simulink model "target_driver_2022_Ctrl_v_2_4_landing_2017a"  (R2024b)
settings: Solver=FixedStepDiscrete  StartTime=0.0  StopTime=13  FixedStep=0.0001  RelTol=1e-3  EnableMultiTasking=on
values from neighbouring files (symbols this model uses):
  A = gamma_2*gamma_3*Thrust_desired    [force2voltage.m]
  a2_lb = -0.25    [target_driver_setup_2022_Ctrl_V_2_4.m]    (also in target_driver_setup_2022_Ctrl_V_2_4_geometric.m; target_driver_setup_mpc_12msdelay.m; target_driver_setup_mpc_andWLQP.m)
  a2_openloop = -0    (= 0)    [target_driver_setup_2022_Ctrl_V_2_4.m]    (also in target_driver_setup_2022_Ctrl_V_2_4_geometric.m; target_driver_setup_mpc_12msdelay.m; target_driver_setup_mpc_andWLQP.m)
  a2_ub = 0.25    [target_driver_setup_2022_Ctrl_V_2_4.m]    (also in target_driver_setup_2022_Ctrl_V_2_4_geometric.m; target_driver_setup_mpc_12msdelay.m; target_driver_setup_mpc_andWLQP.m)
  adaptive_flag = 0    [target_driver_setup_2022_Ctrl_V_2_4.m]    (also in target_driver_setup_2022_Ctrl_V_2_4_geometric.m; target_driver_setup_mpc_12msdelay.m = 1; target_driver_setup_mpc_andWLQP.m = 1)
  adaptive_gain = [gamma_adaptive, adaptive_roll_limit, adaptive_pitch_limit, adaptive_yaw_limit, c_2_adaptive, gamma_lateral_adaptive, adaptive_x_limit, adaptive_y_limit, adaptive_z_limit, c_1_adaptive]    [target_driver_setup_2022_Ctrl_V_2_4.m]    (also in target_driver_setup_2022_Ctrl_V_2_4_geometric.m; target_driver_setup_mpc_12msdelay.m; target_driver_setup_mpc_andWLQP.m)
  adaptive_lateral_flag = 0    [target_driver_setup_2022_Ctrl_V_2_4.m]    (also in target_driver_setup_2022_Ctrl_V_2_4_geometric.m; target_driver_setup_mpc_12msdelay.m = 1; target_driver_setup_mpc_andWLQP.m = 1)
  adaptive_pitch_init = 0    [target_driver_setup_2022_Ctrl_V_2_4.m]    (also in target_driver_setup_2022_Ctrl_V_2_4_geometric.m; target_driver_setup_mpc_12msdelay.m; target_driver_setup_mpc_andWLQP.m)
  adaptive_pitch_limit = 0.1/(scale^2)    (= 1e-07)    [target_driver_setup_2022_Ctrl_V_2_4.m]    (also in target_driver_setup_2022_Ctrl_V_2_4_geometric.m = 3e-07; target_driver_setup_mpc_12msdelay.m; target_driver_setup_mpc_andWLQP.m)
  adaptive_pitch_limit_low = -adaptive_pitch_limit    (= -1e-07)    [target_driver_setup_2022_Ctrl_V_2_4.m]    (also in target_driver_setup_2022_Ctrl_V_2_4_geometric.m = -3e-07; target_driver_setup_mpc_12msdelay.m; target_driver_setup_mpc_andWLQP.m)
  adaptive_roll_init = 0    [target_driver_setup_2022_Ctrl_V_2_4.m]    (also in target_driver_setup_2022_Ctrl_V_2_4_geometric.m; target_driver_setup_mpc_12msdelay.m; target_driver_setup_mpc_andWLQP.m)
  adaptive_roll_limit = 0.3/(scale^2)    (= 3e-07)    [target_driver_setup_2022_Ctrl_V_2_4.m]    (also in target_driver_setup_2022_Ctrl_V_2_4_geometric.m; target_driver_setup_mpc_12msdelay.m; target_driver_setup_mpc_andWLQP.m)
  adaptive_roll_limit_low = -adaptive_roll_limit    (= -3e-07)    [target_driver_setup_2022_Ctrl_V_2_4.m]    (also in target_driver_setup_2022_Ctrl_V_2_4_geometric.m; target_driver_setup_mpc_12msdelay.m; target_driver_setup_mpc_andWLQP.m)
  adaptive_x_init = 0    [target_driver_setup_2022_Ctrl_V_2_4.m]    (also in target_driver_setup_2022_Ctrl_V_2_4_geometric.m; target_driver_setup_mpc_12msdelay.m; target_driver_setup_mpc_andWLQP.m)
  adaptive_x_limit = 0.15/(scale)    (= 0.00015)    [target_driver_setup_2022_Ctrl_V_2_4.m]    (also in target_driver_setup_2022_Ctrl_V_2_4_geometric.m = 7.5e-05; target_driver_setup_mpc_12msdelay.m; target_driver_setup_mpc_andWLQP.m)
  adaptive_x_limit_low = -adaptive_x_limit    (= -0.00015)    [target_driver_setup_2022_Ctrl_V_2_4.m]    (also in target_driver_setup_2022_Ctrl_V_2_4_geometric.m = -7.5e-05; target_driver_setup_mpc_12msdelay.m; target_driver_setup_mpc_andWLQP.m)
  adaptive_y_init = 0    [target_driver_setup_2022_Ctrl_V_2_4.m]    (also in target_driver_setup_2022_Ctrl_V_2_4_geometric.m; target_driver_setup_mpc_12msdelay.m; target_driver_setup_mpc_andWLQP.m)
  adaptive_y_limit = 0.15/(scale)    (= 0.00015)    [target_driver_setup_2022_Ctrl_V_2_4.m]    (also in target_driver_setup_2022_Ctrl_V_2_4_geometric.m = 7.5e-05; target_driver_setup_mpc_12msdelay.m; target_driver_setup_mpc_andWLQP.m)
  adaptive_y_limit_low = -adaptive_y_limit    (= -0.00015)    [target_driver_setup_2022_Ctrl_V_2_4.m]    (also in target_driver_setup_2022_Ctrl_V_2_4_geometric.m = -7.5e-05; target_driver_setup_mpc_12msdelay.m; target_driver_setup_mpc_andWLQP.m)
  adaptive_yaw_init = 0    [target_driver_setup_2022_Ctrl_V_2_4.m]    (also in target_driver_setup_2022_Ctrl_V_2_4_geometric.m; target_driver_setup_mpc_12msdelay.m; target_driver_setup_mpc_andWLQP.m)
  adaptive_yaw_limit = 0.035/(scale^2)    (= 3.5e-08)    [target_driver_setup_2022_Ctrl_V_2_4.m]    (also in target_driver_setup_2022_Ctrl_V_2_4_geometric.m; target_driver_setup_mpc_12msdelay.m; target_driver_setup_mpc_andWLQP.m)
  adaptive_yaw_limit_low = -adaptive_yaw_limit    (= -3.5e-08)    [target_driver_setup_2022_Ctrl_V_2_4.m]    (also in target_driver_setup_2022_Ctrl_V_2_4_geometric.m; target_driver_setup_mpc_12msdelay.m; target_driver_setup_mpc_andWLQP.m)
  adaptive_z_init = 0/scale    (= 0)    [target_driver_setup_2022_Ctrl_V_2_4.m]    (also in target_driver_setup_2022_Ctrl_V_2_4_geometric.m; target_driver_setup_mpc_12msdelay.m; target_driver_setup_mpc_andWLQP.m)
  adaptive_z_limit = 0.20/(scale)    (= 0.0002)    [target_driver_setup_2022_Ctrl_V_2_4.m]    (also in target_driver_setup_2022_Ctrl_V_2_4_geometric.m = 0.0008; target_driver_setup_mpc_12msdelay.m = 0.0008; target_driver_setup_mpc_andWLQP.m = 0.0008)
  adaptive_z_limit_low = -adaptive_z_limit/1    (= -0.0002)    [target_driver_setup_2022_Ctrl_V_2_4.m]    (also in target_driver_setup_2022_Ctrl_V_2_4_geometric.m = -0.0008; target_driver_setup_mpc_12msdelay.m = -0.0008; target_driver_setup_mpc_andWLQP.m = -0.0008)
  att_s = 500    [target_driver_setup_2022_Ctrl_V_2_4.m]    (also in target_driver_setup_2022_Ctrl_V_2_4_geometric.m; target_driver_setup_mpc_12msdelay.m; target_driver_setup_mpc_andWLQP.m)
  b_1_d_desired = [1,0,0]    [target_driver_setup_2022_Ctrl_V_2_4.m]    (also in target_driver_setup_2022_Ctrl_V_2_4_geometric.m; target_driver_setup_mpc_12msdelay.m; target_driver_setup_mpc_andWLQP.m)
  closedloop_flag = 1    [target_driver_setup_2022_Ctrl_V_2_4.m]    (also in target_driver_setup_2022_Ctrl_V_2_4_geometric.m = 0; target_driver_setup_mpc_12msdelay.m = 0; target_driver_setup_mpc_andWLQP.m = 0)
  control_gain = [k_x,k_v, k_R, k_Omega, k_z, k_vz, k_Rx]    [target_driver_setup_2022_Ctrl_V_2_4.m]    (also in target_driver_setup_2022_Ctrl_V_2_4_geometric.m = [k_x,k_v,k_R,k_Omega_pitch,k_Omega_roll,k_z,k_vz,k_Rx]; target_driver_setup_mpc_12msdelay.m = [k_x, k_v, k_R, k_Omega, k_z, k_vz, k_Rx,                  k; target_driver_setup_mpc_andWLQP.m = [k_x, k_v, k_R, k_Omega, k_z, k_vz, k_Rx,                  k)
  delay = delay-vicon_sample_cycle/2    [target_driver_setup_2022_Ctrl_V_2_4.m]    (also in target_driver_setup_2022_Ctrl_V_2_4_geometric.m; target_driver_setup_mpc_12msdelay.m; target_driver_setup_mpc_andWLQP.m)
  drv_amp = abs((vleft_p2p-vright_p2p))/2+min(vleft_p2p,vright_p2p)    [Wing_traj_to_Voltage.m]    (also in force2voltage.m; target_driver_setup_2022_Ctrl_V_2_4.m = 160; target_driver_setup_2022_Ctrl_V_2_4_geometric.m = 110; target_driver_setup_mpc_12msdelay.m = 150)
  drv_bias = max_drv_bias    (= 300)    [target_driver_setup_2022_Ctrl_V_2_4.m]    (also in target_driver_setup_2022_Ctrl_V_2_4_geometric.m = 200; target_driver_setup_mpc_12msdelay.m = 200; target_driver_setup_mpc_andWLQP.m = 200)
  drv_pitch_left = vleft_pitch    [Wing_traj_to_Voltage.m]    (also in force2voltage.m = 0; target_driver_setup_2022_Ctrl_V_2_4.m = 0; target_driver_setup_2022_Ctrl_V_2_4_geometric.m = 9.05; target_driver_setup_mpc_12msdelay.m = 9.05)
  drv_pitch_right = vright_pitch    [Wing_traj_to_Voltage.m]    (also in force2voltage.m = 0; target_driver_setup_2022_Ctrl_V_2_4.m = 0; target_driver_setup_2022_Ctrl_V_2_4_geometric.m = 9.05; target_driver_setup_mpc_12msdelay.m = 9.05)
  drv_roll = (vleft_p2p-vright_p2p)/4    [Wing_traj_to_Voltage.m]    (also in force2voltage.m; target_driver_setup_2022_Ctrl_V_2_4.m = -2; target_driver_setup_2022_Ctrl_V_2_4_geometric.m = -0.001; target_driver_setup_mpc_12msdelay.m = -0.001)
  f_fin = f    (= 155)    [target_driver_setup_2022_Ctrl_V_2_4.m]    (also in target_driver_setup_2022_Ctrl_V_2_4_geometric.m; target_driver_setup_mpc_12msdelay.m; target_driver_setup_mpc_andWLQP.m)
  f_int = f    (= 155)    [target_driver_setup_2022_Ctrl_V_2_4.m]    (also in target_driver_setup_2022_Ctrl_V_2_4_geometric.m; target_driver_setup_mpc_12msdelay.m; target_driver_setup_mpc_andWLQP.m)
  g = 9.8    [target_driver_setup_2022_Ctrl_V_2_4.m]    (also in target_driver_setup_2022_Ctrl_V_2_4_geometric.m; target_driver_setup_mpc_12msdelay.m; target_driver_setup_mpc_andWLQP.m = 9.81; test_full_attitude_mpc.m = 9.81)
  I_moment_vec = [Ixx, Iyy, Izz]    [target_driver_setup_2022_Ctrl_V_2_4.m]    (also in target_driver_setup_2022_Ctrl_V_2_4_geometric.m; target_driver_setup_mpc_12msdelay.m; target_driver_setup_mpc_andWLQP.m)
  landing_flag = 0    [target_driver_setup_2022_Ctrl_V_2_4.m]    (also in target_driver_setup_2022_Ctrl_V_2_4_geometric.m; target_driver_setup_mpc_12msdelay.m; target_driver_setup_mpc_andWLQP.m)
  landing_parameter = [start_delay+T,transition_rate, rising_time, falling_time, landing_rising_time, landing_z_decrease, landing_y_decrease, landing_x_decrease]    [target_driver_setup_2022_Ctrl_V_2_4.m]    (also in target_driver_setup_2022_Ctrl_V_2_4_geometric.m; target_driver_setup_mpc_12msdelay.m; target_driver_setup_mpc_andWLQP.m)
  low_bound = -8    [target_driver_setup_2022_Ctrl_V_2_4.m]    (also in target_driver_setup_2022_Ctrl_V_2_4_geometric.m = -5; target_driver_setup_mpc_12msdelay.m = -10; target_driver_setup_mpc_andWLQP.m = -10)
  low_bound_eR = -0.8    [target_driver_setup_2022_Ctrl_V_2_4.m]    (also in target_driver_setup_2022_Ctrl_V_2_4_geometric.m = -1.2; target_driver_setup_mpc_12msdelay.m = -1.2; target_driver_setup_mpc_andWLQP.m = -1.2)
  low_bound_vx = -0.5    [target_driver_setup_2022_Ctrl_V_2_4.m]    (also in target_driver_setup_2022_Ctrl_V_2_4_geometric.m; target_driver_setup_mpc_12msdelay.m; target_driver_setup_mpc_andWLQP.m)
  low_bound_vy = -0.5    [target_driver_setup_2022_Ctrl_V_2_4.m]    (also in target_driver_setup_2022_Ctrl_V_2_4_geometric.m; target_driver_setup_mpc_12msdelay.m; target_driver_setup_mpc_andWLQP.m)
  low_bound_vz = -0.5    [target_driver_setup_2022_Ctrl_V_2_4.m]    (also in target_driver_setup_2022_Ctrl_V_2_4_geometric.m; target_driver_setup_mpc_12msdelay.m; target_driver_setup_mpc_andWLQP.m)
  low_bound_x = -0.06    [target_driver_setup_2022_Ctrl_V_2_4.m]    (also in target_driver_setup_2022_Ctrl_V_2_4_geometric.m = -0.1; target_driver_setup_mpc_12msdelay.m = -0.6; target_driver_setup_mpc_andWLQP.m = -0.6)
  low_bound_y = -0.06    [target_driver_setup_2022_Ctrl_V_2_4.m]    (also in target_driver_setup_2022_Ctrl_V_2_4_geometric.m; target_driver_setup_mpc_12msdelay.m = -0.6; target_driver_setup_mpc_andWLQP.m = -0.6)
  low_bound_z = -0.04    [target_driver_setup_2022_Ctrl_V_2_4.m]    (also in target_driver_setup_2022_Ctrl_V_2_4_geometric.m; target_driver_setup_mpc_12msdelay.m = -0.1; target_driver_setup_mpc_andWLQP.m = -0.1)
  m = t <= t_zoom    [plot_roll_torque_cmd_vs_actual.m]    (also in plot_roll_torque_cmd_vs_actual_flightlog.m = t >= t0 & t <= t1; target_driver_setup_2022_Ctrl_V_2_4.m = 0.000124; target_driver_setup_2022_Ctrl_V_2_4_geometric.m = 8.5655e-05; target_driver_setup_mpc_12msdelay.m = 8.5655e-05)
  params_vec = [params_opt.delta_1, params_opt.delta_2, params_opt.delta_3,      params_opt.gamma_1, params_opt.gamma_2_1, params_opt.gamma_3,      params_opt.eta, params_opt.nu, params_opt.mu]'    [force2voltage_tuningSandbox.m]    (also in target_driver_setup_2022_Ctrl_V_2_4.m = [params_opt.delta_1, params_opt.delta_2, params_opt.delta_3,; target_driver_setup_2022_Ctrl_V_2_4_geometric.m = [params_opt.delta_1, params_opt.delta_2, params_opt.delta_3,; target_driver_setup_mpc_12msdelay.m = [params_opt.delta_1, params_opt.delta_2, params_opt.delta_3,; target_driver_setup_mpc_andWLQP.m = [params_opt.delta_1, params_opt.delta_2, params_opt.delta_3,)
  phase = 0    [target_driver_setup_2022_Ctrl_V_2_4.m]    (also in target_driver_setup_2022_Ctrl_V_2_4_geometric.m; target_driver_setup_mpc_12msdelay.m; target_driver_setup_mpc_andWLQP.m)
  r_desired = [default_x, default_y,z_desired]    [target_driver_setup_2022_Ctrl_V_2_4.m]    (also in target_driver_setup_2022_Ctrl_V_2_4_geometric.m; target_driver_setup_mpc_12msdelay.m; target_driver_setup_mpc_andWLQP.m)
  roll_offset_angle = 0    [target_driver_setup_2022_Ctrl_V_2_4.m]    (also in target_driver_setup_2022_Ctrl_V_2_4_geometric.m; target_driver_setup_mpc_12msdelay.m; target_driver_setup_mpc_andWLQP.m)
  running_time = start_delay+total_T    (= 8.5)    [target_driver_setup_2022_Ctrl_V_2_4.m]    (also in target_driver_setup_2022_Ctrl_V_2_4_geometric.m = 10; target_driver_setup_mpc_12msdelay.m = 0.5; target_driver_setup_mpc_andWLQP.m = 10)
  running_time_control = start_delay_control+total_T+0.0    (= 8.6)    [target_driver_setup_2022_Ctrl_V_2_4.m]    (also in target_driver_setup_2022_Ctrl_V_2_4_geometric.m = 10; target_driver_setup_mpc_12msdelay.m = 0.5; target_driver_setup_mpc_andWLQP.m = 10)
  start_delay = 2.0    (= 2)    [target_driver_setup_2022_Ctrl_V_2_4.m]    (also in target_driver_setup_2022_Ctrl_V_2_4_geometric.m = 0; target_driver_setup_mpc_12msdelay.m = 0; target_driver_setup_mpc_andWLQP.m = 0)
  start_delay_control = start_delay + ramp_delay    (= 2.1)    [target_driver_setup_2022_Ctrl_V_2_4.m]    (also in target_driver_setup_2022_Ctrl_V_2_4_geometric.m = 0; target_driver_setup_mpc_12msdelay.m = 0; target_driver_setup_mpc_andWLQP.m = 0)
  T = 0.5    [target_driver_setup_2022_Ctrl_V_2_4.m]    (also in target_driver_setup_2022_Ctrl_V_2_4_geometric.m = 10; target_driver_setup_mpc_12msdelay.m; target_driver_setup_mpc_andWLQP.m = 10; test_full_attitude_mpc.m = T0 + nu(1))
  task_flag = 0    [target_driver_setup_2022_Ctrl_V_2_4.m]    (also in target_driver_setup_2022_Ctrl_V_2_4_geometric.m; target_driver_setup_mpc_12msdelay.m; target_driver_setup_mpc_andWLQP.m)
  task_parameter = [radius_ref, frequency_ref, radius_ratio, lissajous_ratio, lissajous_delta, lissajous_amplitude_ratio,z_radius_ratio]    [target_driver_setup_2022_Ctrl_V_2_4.m]    (also in target_driver_setup_2022_Ctrl_V_2_4_geometric.m; target_driver_setup_mpc_12msdelay.m; target_driver_setup_mpc_andWLQP.m)
  upp_bound = 8    [target_driver_setup_2022_Ctrl_V_2_4.m]    (also in target_driver_setup_2022_Ctrl_V_2_4_geometric.m = 5; target_driver_setup_mpc_12msdelay.m = 10; target_driver_setup_mpc_andWLQP.m = 10)
  upp_bound_eR = 0.8    [target_driver_setup_2022_Ctrl_V_2_4.m]    (also in target_driver_setup_2022_Ctrl_V_2_4_geometric.m = 1.2; target_driver_setup_mpc_12msdelay.m = 1.2; target_driver_setup_mpc_andWLQP.m = 1.2)
  upp_bound_vx = 0.5    [target_driver_setup_2022_Ctrl_V_2_4.m]    (also in target_driver_setup_2022_Ctrl_V_2_4_geometric.m; target_driver_setup_mpc_12msdelay.m; target_driver_setup_mpc_andWLQP.m)
  upp_bound_vy = 0.5    [target_driver_setup_2022_Ctrl_V_2_4.m]    (also in target_driver_setup_2022_Ctrl_V_2_4_geometric.m; target_driver_setup_mpc_12msdelay.m; target_driver_setup_mpc_andWLQP.m)
  upp_bound_vz = 0.5    [target_driver_setup_2022_Ctrl_V_2_4.m]    (also in target_driver_setup_2022_Ctrl_V_2_4_geometric.m; target_driver_setup_mpc_12msdelay.m; target_driver_setup_mpc_andWLQP.m)
  upp_bound_x = 0.06    [target_driver_setup_2022_Ctrl_V_2_4.m]    (also in target_driver_setup_2022_Ctrl_V_2_4_geometric.m = 0.1; target_driver_setup_mpc_12msdelay.m = 0.6; target_driver_setup_mpc_andWLQP.m = 0.6)
  upp_bound_y = 0.06    [target_driver_setup_2022_Ctrl_V_2_4.m]    (also in target_driver_setup_2022_Ctrl_V_2_4_geometric.m; target_driver_setup_mpc_12msdelay.m = 0.6; target_driver_setup_mpc_andWLQP.m = 0.6)
  upp_bound_z = 0.04    [target_driver_setup_2022_Ctrl_V_2_4.m]    (also in target_driver_setup_2022_Ctrl_V_2_4_geometric.m; target_driver_setup_mpc_12msdelay.m = 0.1; target_driver_setup_mpc_andWLQP.m = 0.1)
undefined symbols (not defined in the file or in its folder): Com1, DiscIntNeverNeededParam, left_mapping, left_mapping_F_to_Phi, lp_den, lp_num, none, right_mapping, right_mapping_F_to_Phi, vlp_den, vlp_num
libraries: simulink x32, xpcseriallib x6, xpcnilib x3, xpcutilitieslib x3
(part 2 of 7)

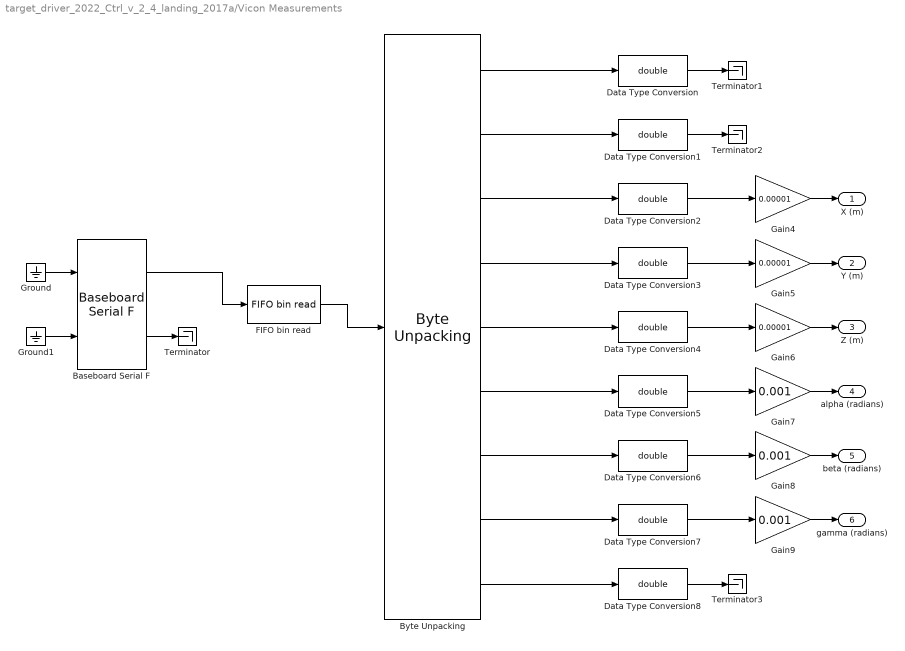
== system target_driver_2022_Ctrl_v_2_4_landing_2017a/Vicon Measurements ==
  Baseboard Serial F : xpcseriallib/Mainboard/Baseboard Serial F  group=FIFO Setup  port=1  irqnum=4  saddr1=0x3f8  saddr2=0x3e8  config=Com1/none  baud1=115200  parity1=None  ndata1=8  nstop1=1  fifomode1=16 deep  rlevel1=half full  automode1=on  xmtfifosize1=1024  xmtdatatype1=8 bit int null terminated  rcvfifosize1=1024  baud2=115200  parity2=None  ndata2=8  nstop2=1  fifomode2=16 deep  rlevel2=half full  automode2=off  xmtfifosize2=1024  xmtdatatype2=8 bit uint null terminated  rcvfifosize2=1024
      settings: SourceProductName=Simulink Real-Time
  "Byte Unpacking " : xpcutilitieslib/Byte Unpacking   MaskUnpackedDataTypes={'uint8','int16','int16','int16','int16','int16','int16','int16','uint8'}  MaskUnpackedDataSizes={[1] [1] [1] [1] [1] [1] [1] [1] [1]}  MaskAlignment=1
      settings: SourceProductName=Simulink Real-Time
  Data Type Conversion{,1..8} (9 alike) : DataTypeConversion  OutDataTypeStr=double  SaturateOnIntegerOverflow=off  RndMeth=Floor
  "FIFO bin read " : xpcseriallib/FIFO bin read   header=[128,127,127]  lengths=[15]  hold=Hold last output if no new data  enable=off  maxsize=15  outputtype=8 bit uint null terminated  sampletime=0.0001
      settings: SourceProductName=Simulink Real-Time
  Gain4 : Gain  Gain=0.00001
  Gain5 : Gain  Gain=0.00001
  Gain6 : Gain  Gain=0.00001
  Gain7 : Gain  Gain=0.001
  Gain8 : Gain  Gain=0.001
  Gain9 : Gain  Gain=0.001
  Ground : Ground
  Ground1 : Ground
  Terminator{,1..3} (4 alike) : Terminator
  X (m) : Outport
  Y (m) : Outport  Port=2
  Z (m) : Outport  Port=3
  alpha (radians) : Outport  Port=4
  beta (radians) : Outport  Port=5
  gamma (radians) : Outport  Port=6
  wires:
  Baseboard Serial F/1 -> "FIFO bin read "/1
  Baseboard Serial F/2 -> Terminator/1
  Ground1/1 -> Baseboard Serial F/2
  Ground/1 -> Baseboard Serial F/1
  "Byte Unpacking "/1 -> Data Type Conversion/1
  "Byte Unpacking "/2 -> Data Type Conversion1/1
  "Byte Unpacking "/3 -> Data Type Conversion2/1
  "Byte Unpacking "/4 -> Data Type Conversion3/1
  "FIFO bin read "/1 -> "Byte Unpacking "/1
  "Byte Unpacking "/8 -> Data Type Conversion7/1
  "Byte Unpacking "/7 -> Data Type Conversion6/1
  "Byte Unpacking "/5 -> Data Type Conversion4/1
  "Byte Unpacking "/6 -> Data Type Conversion5/1
  Data Type Conversion3/1 -> Gain5/1
  Data Type Conversion4/1 -> Gain6/1
  Data Type Conversion5/1 -> Gain7/1
  Data Type Conversion6/1 -> Gain8/1
  Data Type Conversion7/1 -> Gain9/1
  "Byte Unpacking "/9 -> Data Type Conversion8/1
  Gain4/1 -> X (m)/1
  Data Type Conversion2/1 -> Gain4/1
  Gain5/1 -> Y (m)/1
  Gain6/1 -> Z (m)/1
  Gain7/1 -> alpha (radians)/1
  Gain8/1 -> beta (radians)/1
  Gain9/1 -> gamma (radians)/1
  Data Type Conversion/1 -> Terminator1/1
  Data Type Conversion1/1 -> Terminator2/1
  Data Type Conversion8/1 -> Terminator3/1

== system target_driver_2022_Ctrl_v_2_4_landing_2017a/Vicon Post Processing ==
  note: Process Vicon data
      |
      | 1) Generate Raw rotation matrix
      | 2) Flag the update of new vicon data
      | 3) Count the number of samples before new update
      |
      | By Patrick 2021 Mar
  alpha : Inport
  beta : Inport  Port=2
  gamma : Inport  Port=3
  Raw rotation matrix : Subsystem
  Vicon Validity check : Subsystem
  Vicon correction : MATLAB Function  TreatAsAtomicUnit=on
  roll_offset_angle : Constant  Value=roll_offset_angle  SampleTime=-1
  "Vicon Update Flag " : Outport
  Raw Rotation Matrix : Outport  Port=2
  "Vicon Count " : Outport  Port=3
  wires:
  Vicon Validity check/2(Vicon Count) -> "Vicon Count "/1
  beta/1 -> Raw rotation matrix/2(beta)
  gamma/1 -> Raw rotation matrix/3(gamma)
  alpha/1 -> Raw rotation matrix/1(alpha)
  Vicon Validity check/1("Vicon Update flag ") -> "Vicon Update Flag "/1
  roll_offset_angle/1 -> Vicon correction/2(roll_offset_angle)
  Raw rotation matrix/1(R) -> Vicon correction/1(R_cur)
  Vicon correction/1(Rot_corrected_vec) -> Raw Rotation Matrix/1, Vicon Validity check/1("Rotation Matrix ")

== system target_driver_2022_Ctrl_v_2_4_landing_2017a/Vicon Post Processing1 ==
  note: Process Vicon data
      |
      | 1) Generate Raw rotation matrix
      | 2) Flag the update of new vicon data
      | 3) Count the number of samples before new update
      |
      | By Patrick 2021 Mar
  alpha : Inport
  beta : Inport  Port=2
  gamma : Inport  Port=3
  Raw rotation matrix : Subsystem
  Vicon Validity check : Subsystem
  Vicon correction : MATLAB Function  TreatAsAtomicUnit=on
  roll_offset_angle : Constant  Value=roll_offset_angle  SampleTime=-1
  "Vicon Update Flag " : Outport
  Raw Rotation Matrix : Outport  Port=2
  "Vicon Count " : Outport  Port=3
  wires:
  Vicon Validity check/2(Vicon Count) -> "Vicon Count "/1
  beta/1 -> Raw rotation matrix/2(beta)
  gamma/1 -> Raw rotation matrix/3(gamma)
  alpha/1 -> Raw rotation matrix/1(alpha)
  Vicon Validity check/1("Vicon Update flag ") -> "Vicon Update Flag "/1
  roll_offset_angle/1 -> Vicon correction/2(roll_offset_angle)
  Raw rotation matrix/1(R) -> Vicon correction/1(R_cur)
  Vicon correction/1(Rot_corrected_vec) -> Raw Rotation Matrix/1, Vicon Validity check/1("Rotation Matrix ")

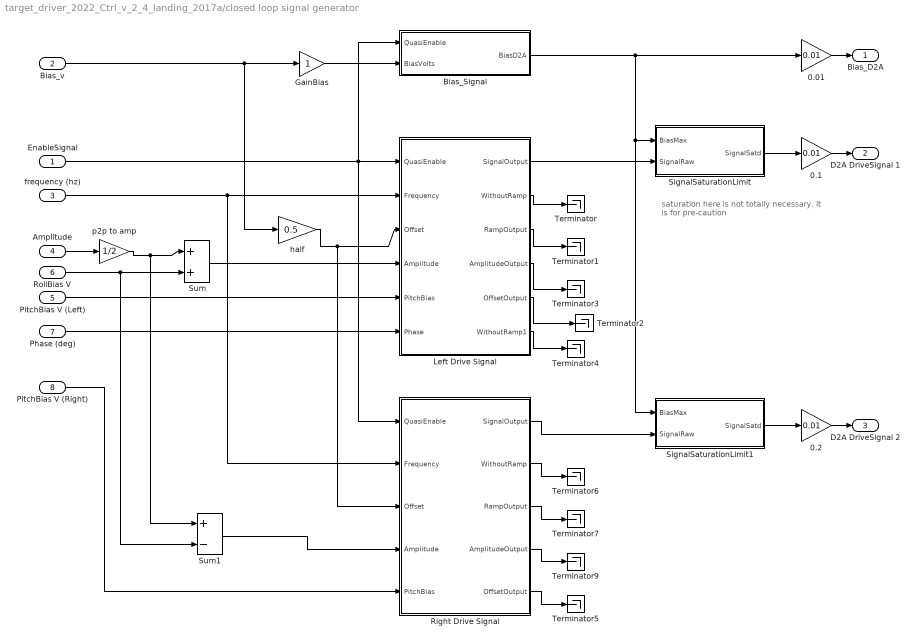
== system target_driver_2022_Ctrl_v_2_4_landing_2017a/closed loop signal generator ==
  note: saturation here is not totally necessary.
      | it is for pre-caution
  EnableSignal : Inport
  Bias_v : Inport  Port=2
  frequency (hz) : Inport  Port=3
  Amplitude : Inport  Port=4
  PitchBias V (Left) : Inport  Port=5
  RollBias V : Inport  Port=6
  Phase (deg) : Inport  Port=7
  PitchBias V (Right) : Inport  Port=8
  0.01 : Gain  Gain=0.01
  0.1 : Gain  Gain=0.01
  0.2 : Gain  Gain=0.01
  Bias_Signal : Subsystem
  GainBias : Gain
  "Left Drive Signal " : Subsystem
  Right Drive Signal : Subsystem
  SignalSaturationLimit : Subsystem
  SignalSaturationLimit1 : Subsystem
  Sum : Sum
  Sum1 : Sum  Inputs=+-
  Terminator{,1..7,9} (9 alike) : Terminator
  half : Gain  Gain=0.5
  p2p to amp : Gain  Gain=1/2
  Bias_D2A : Outport
  D2A DriveSignal 1 : Outport  Port=2
  D2A DriveSignal 2 : Outport  Port=3
  wires:
  Bias_Signal/1(BiasD2A) -> SignalSaturationLimit1/1(BiasMax), SignalSaturationLimit/1(BiasMax), 0.01/1
  half/1 -> "Left Drive Signal "/3(Offset), Right Drive Signal/3(Offset)
  Bias_v/1 -> GainBias/1, half/1
  EnableSignal/1 -> "Left Drive Signal "/1(QuasiEnable), Bias_Signal/1(QuasiEnable), Right Drive Signal/1(QuasiEnable)
  frequency (hz)/1 -> Right Drive Signal/2(Frequency), "Left Drive Signal "/2(Frequency)
  "Left Drive Signal "/2(WithoutRamp) -> Terminator/1
  "Left Drive Signal "/3(RampOutput) -> Terminator1/1
  "Left Drive Signal "/5(OffsetOutput) -> Terminator2/1
  SignalSaturationLimit/1(SignalSatd) -> 0.1/1
  GainBias/1 -> Bias_Signal/2(BiasVolts)
  Sum/1 -> "Left Drive Signal "/4(Amplitude)
  RollBias V/1 -> Sum/2, Sum1/2
  SignalSaturationLimit1/1(SignalSatd) -> 0.2/1
  Right Drive Signal/5(OffsetOutput) -> Terminator5/1
  Amplitude/1 -> p2p to amp/1
  p2p to amp/1 -> Sum/1, Sum1/1
  "Left Drive Signal "/4(AmplitudeOutput) -> Terminator3/1
  Right Drive Signal/2(WithoutRamp) -> Terminator6/1
  Right Drive Signal/3(RampOutput) -> Terminator7/1
  Right Drive Signal/4(AmplitudeOutput) -> Terminator9/1
  0.01/1 -> Bias_D2A/1
  0.1/1 -> D2A DriveSignal 1/1
  0.2/1 -> D2A DriveSignal 2/1
  Sum1/1 -> Right Drive Signal/4(Amplitude)
  Right Drive Signal/1(SignalOutput) -> SignalSaturationLimit1/2(SignalRaw)
  "Left Drive Signal "/1(SignalOutput) -> SignalSaturationLimit/2(SignalRaw)
  Phase (deg)/1 -> "Left Drive Signal "/6(Phase)
  "Left Drive Signal "/6(WithoutRamp1) -> Terminator4/1
  PitchBias V (Left)/1 -> "Left Drive Signal "/5(PitchBias)
  PitchBias V (Right)/1 -> Right Drive Signal/5(PitchBias)

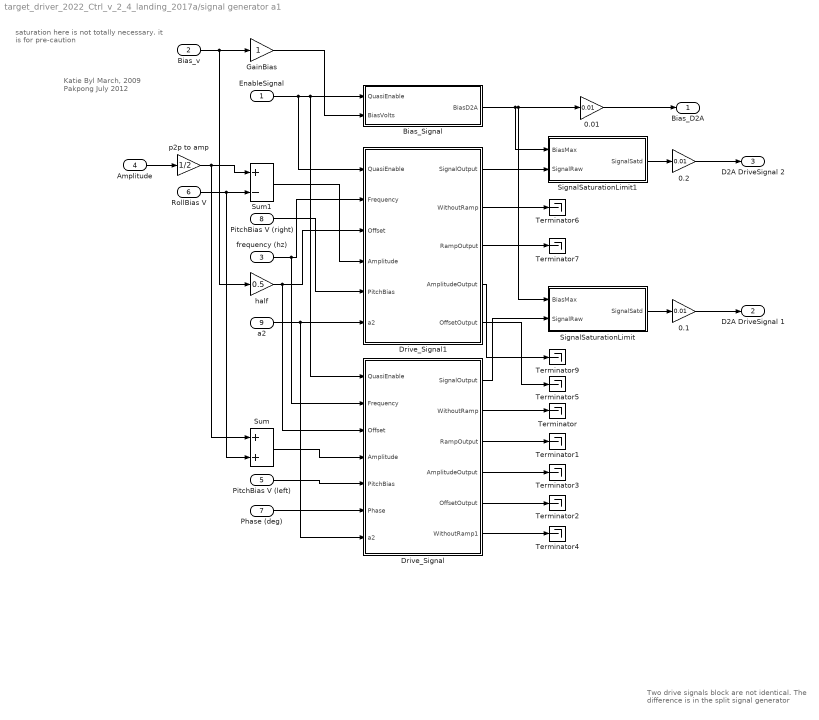
== system target_driver_2022_Ctrl_v_2_4_landing_2017a/signal generator a1 ==
  note: Katie Byl
      | March, 2009
      |
      | Pakpong
      | July 2012
  note: Two drive signals block are not identical.
      | The difference is in the split signal generator
  note: saturation here is not totally necessary.
      | it is for pre-caution
  EnableSignal : Inport
  Bias_v : Inport  Port=2
  frequency (hz) : Inport  Port=3
  Amplitude : Inport  Port=4
  PitchBias V (left) : Inport  Port=5
  RollBias V : Inport  Port=6
  Phase (deg) : Inport  Port=7
  PitchBias V (right) : Inport  Port=8
  a2 : Inport  Port=9
  0.01 : Gain  Gain=0.01
  0.1 : Gain  Gain=0.01
  0.2 : Gain  Gain=0.01
  Bias_Signal : Subsystem
  Drive_Signal : Subsystem
  Drive_Signal1 : Subsystem
  GainBias : Gain
  SignalSaturationLimit : Subsystem
  SignalSaturationLimit1 : Subsystem
  Sum : Sum
  Sum1 : Sum  Inputs=+-
  Terminator{,1..7,9} (9 alike) : Terminator
  half : Gain  Gain=0.5
  p2p to amp : Gain  Gain=1/2
  Bias_D2A : Outport
  D2A DriveSignal 1 : Outport  Port=2
  D2A DriveSignal 2 : Outport  Port=3
  wires:
  0.1/1 -> D2A DriveSignal 1/1
  0.2/1 -> D2A DriveSignal 2/1
  SignalSaturationLimit1/1(SignalSatd) -> 0.2/1
  0.01/1 -> Bias_D2A/1
  SignalSaturationLimit/1(SignalSatd) -> 0.1/1
  Drive_Signal/5(OffsetOutput) -> Terminator2/1
  GainBias/1 -> Bias_Signal/2(BiasVolts)
  Drive_Signal/1(SignalOutput) -> SignalSaturationLimit/2(SignalRaw)
  Drive_Signal1/5(OffsetOutput) -> Terminator5/1
  half/1 -> Drive_Signal1/3(Offset), Drive_Signal/3(Offset)
  Drive_Signal1/4(AmplitudeOutput) -> Terminator9/1
  Drive_Signal1/3(RampOutput) -> Terminator7/1
  PitchBias V (left)/1 -> Drive_Signal/5(PitchBias)
  Bias_Signal/1(BiasD2A) -> 0.01/1, SignalSaturationLimit/1(BiasMax), SignalSaturationLimit1/1(BiasMax)
  Drive_Signal1/2(WithoutRamp) -> Terminator6/1
  Drive_Signal/6(WithoutRamp1) -> Terminator4/1
  a2/1 -> Drive_Signal1/6(a2), Drive_Signal/7("a2 ")
  Drive_Signal/2(WithoutRamp) -> Terminator/1
  Phase (deg)/1 -> Drive_Signal/6(Phase)
  frequency (hz)/1 -> Drive_Signal/2(Frequency), Drive_Signal1/2(Frequency)
  RollBias V/1 -> Sum1/2, Sum/2
  Sum1/1 -> Drive_Signal1/4(Amplitude)
  Drive_Signal/4(AmplitudeOutput) -> Terminator3/1
  PitchBias V (right)/1 -> Drive_Signal1/5(PitchBias)
  EnableSignal/1 -> Bias_Signal/1(QuasiEnable), Drive_Signal/1(QuasiEnable), Drive_Signal1/1(QuasiEnable)
  Amplitude/1 -> p2p to amp/1
  Sum/1 -> Drive_Signal/4(Amplitude)
  Bias_v/1 -> half/1, GainBias/1
  Drive_Signal/3(RampOutput) -> Terminator1/1
  Drive_Signal1/1(SignalOutput) -> SignalSaturationLimit1/2(SignalRaw)
  p2p to amp/1 -> Sum1/1, Sum/1

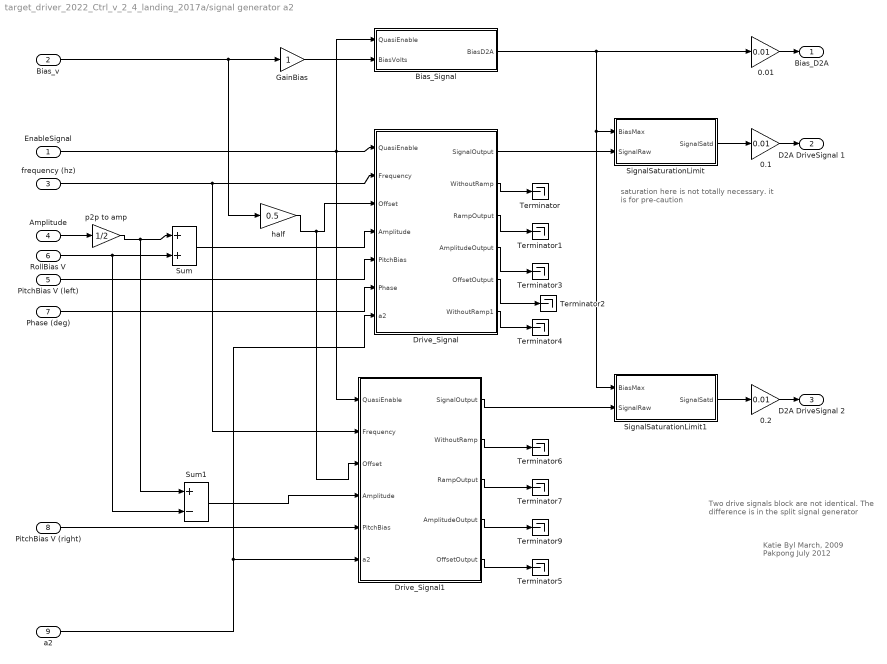
== system target_driver_2022_Ctrl_v_2_4_landing_2017a/signal generator a2 ==
  note: Katie Byl
      | March, 2009
      |
      | Pakpong
      | July 2012
  note: Two drive signals block are not identical.
      | The difference is in the split signal generator
  note: saturation here is not totally necessary.
      | it is for pre-caution
  EnableSignal : Inport
  Bias_v : Inport  Port=2
  frequency (hz) : Inport  Port=3
  Amplitude : Inport  Port=4
  PitchBias V (left) : Inport  Port=5
  RollBias V : Inport  Port=6
  Phase (deg) : Inport  Port=7
  PitchBias V (right) : Inport  Port=8
  a2 : Inport  Port=9
  0.01 : Gain  Gain=0.01
  0.1 : Gain  Gain=0.01
  0.2 : Gain  Gain=0.01
  Bias_Signal : Subsystem
  Drive_Signal : Subsystem
  Drive_Signal1 : Subsystem
  GainBias : Gain
  SignalSaturationLimit : Subsystem
  SignalSaturationLimit1 : Subsystem
  Sum : Sum
  Sum1 : Sum  Inputs=+-
  Terminator{,1..7,9} (9 alike) : Terminator
  half : Gain  Gain=0.5
  p2p to amp : Gain  Gain=1/2
  Bias_D2A : Outport
  D2A DriveSignal 1 : Outport  Port=2
  D2A DriveSignal 2 : Outport  Port=3
  wires:
  Bias_Signal/1(BiasD2A) -> SignalSaturationLimit1/1(BiasMax), SignalSaturationLimit/1(BiasMax), 0.01/1
  half/1 -> Drive_Signal/3(Offset), Drive_Signal1/3(Offset)
  Bias_v/1 -> GainBias/1, half/1
  EnableSignal/1 -> Drive_Signal/1(QuasiEnable), Bias_Signal/1(QuasiEnable), Drive_Signal1/1(QuasiEnable)
  frequency (hz)/1 -> Drive_Signal1/2(Frequency), Drive_Signal/2(Frequency)
  Drive_Signal/2(WithoutRamp) -> Terminator/1
  Drive_Signal/3(RampOutput) -> Terminator1/1
  Drive_Signal/5(OffsetOutput) -> Terminator2/1
  SignalSaturationLimit/1(SignalSatd) -> 0.1/1
  GainBias/1 -> Bias_Signal/2(BiasVolts)
  Sum/1 -> Drive_Signal/4(Amplitude)
  RollBias V/1 -> Sum/2, Sum1/2
  SignalSaturationLimit1/1(SignalSatd) -> 0.2/1
  Drive_Signal1/5(OffsetOutput) -> Terminator5/1
  Amplitude/1 -> p2p to amp/1
  p2p to amp/1 -> Sum/1, Sum1/1
  Drive_Signal/4(AmplitudeOutput) -> Terminator3/1
  Drive_Signal1/2(WithoutRamp) -> Terminator6/1
  Drive_Signal1/3(RampOutput) -> Terminator7/1
  Drive_Signal1/4(AmplitudeOutput) -> Terminator9/1
  0.01/1 -> Bias_D2A/1
  0.1/1 -> D2A DriveSignal 1/1
  0.2/1 -> D2A DriveSignal 2/1
  Sum1/1 -> Drive_Signal1/4(Amplitude)
  Drive_Signal1/1(SignalOutput) -> SignalSaturationLimit1/2(SignalRaw)
  Drive_Signal/1(SignalOutput) -> SignalSaturationLimit/2(SignalRaw)
  Phase (deg)/1 -> Drive_Signal/6(Phase)
  Drive_Signal/6(WithoutRamp1) -> Terminator4/1
  PitchBias V (left)/1 -> Drive_Signal/5(PitchBias)
  a2/1 -> Drive_Signal/7("a2 "), Drive_Signal1/6(a2)
  PitchBias V (right)/1 -> Drive_Signal1/5(PitchBias)

== system target_driver_2022_Ctrl_v_2_4_landing_2017a/timer1 ==
  SaturatingRamp : DiscreteIntegrator  gainval=1  SampleTime=-1  UpperSaturationLimit=1  LowerSaturationLimit=0  ICPrevOutput=DiscIntNeverNeededParam  ICPrevScaledInput=DiscIntNeverNeededParam
  constant : Constant
  time : Outport
  wires:
  SaturatingRamp/1 -> time/1
  constant/1 -> SaturatingRamp/1

== system target_driver_2022_Ctrl_v_2_4_landing_2017a/Desired attitude and normalized error/Geometric derivative for Rd in SO(3) ==
  note: First order geometric derivative Rd in SO(3)
      | Patrick 2021 Mar
  Previous Averaged Rotation M : Inport
  Vicon Count : Inport  Port=2
  Current Averaged Rotation M : Inport  Port=3
  "Vicon Update Flag " : Inport  Port=4
  Demux1 : Demux  Outputs=3
  Demux2 : Demux  Outputs=3
  Discrete Derivative : simulink/Discrete/Discrete Derivative  gainval=1.0  ICPrevScaledInput=0.0  OutMin=[]  OutMax=[]  OutDataType=fixdt(1, 16)  OutScaling=2^-10  DoSatur=off
  "First order geometric derivative in SO(3) " : MATLAB Function  TreatAsAtomicUnit=on
  Mux1 : Mux  Inputs=3
  Mux2 : Mux  Inputs=3
  Previous Omega_d : Delay  DelayLength=1  InitialCondition=0
  filtered derivative1 : Subsystem
  filtered derivative5 : Subsystem
  Filtered Geometric derivative dRd in SO(3) : Outport
  Filtered Geometric derivative ddRd in SO(3)1 : Outport  Port=2
  wires:
  Previous Omega_d/1 -> "First order geometric derivative in SO(3) "/3(omega_d_prev)
  Previous Averaged Rotation M/1 -> "First order geometric derivative in SO(3) "/1(R_prev)
  Demux2/1 -> Mux2/1
  Demux2/2 -> Mux2/2
  filtered derivative5/1(Out1) -> Discrete Derivative/1, Demux2/1
  Mux2/1 -> Filtered Geometric derivative dRd in SO(3)/1
  "First order geometric derivative in SO(3) "/1(omega_d) -> Previous Omega_d/1, filtered derivative5/1(In1)
  Demux2/3 -> Mux2/3
  Current Averaged Rotation M/1 -> "First order geometric derivative in SO(3) "/2(R_cur)
  Vicon Count/1 -> "First order geometric derivative in SO(3) "/5(count)
  "Vicon Update Flag "/1 -> "First order geometric derivative in SO(3) "/4(update)
  Demux1/3 -> Mux1/3
  Mux1/1 -> Filtered Geometric derivative ddRd in SO(3)1/1
  Demux1/2 -> Mux1/2
  filtered derivative1/1(Out1) -> Demux1/1
  Demux1/1 -> Mux1/1
  Discrete Derivative/1 -> filtered derivative1/1(In1)

== system target_driver_2022_Ctrl_v_2_4_landing_2017a/Desired attitude and normalized error/saturated normalized error observation ==
  p : Inport
  v : Inport  Port=2
  R : Inport  Port=3
  omega : Inport  Port=4
  "omega_desired " : Inport  Port=5
  R_desired : Inport  Port=6
  r_desired : Inport  Port=7
  "v_desired " : Inport  Port=8
  "Saturated angular velocity eOmega " : Subsystem
  Saturated normalized eR : Subsystem
  "saturated normalized altitude error " : Subsystem
  "Normalized omega error " : Outport
  Normalized eR : Outport  Port=2
  "Normalized position error " : Outport  Port=3
  Normalized velocity error : Outport  Port=4
  wires:
  omega/1 -> "Saturated angular velocity eOmega "/1(omega)
  v/1 -> "saturated normalized altitude error "/1(averaged velocity)
  p/1 -> "saturated normalized altitude error "/2(averaged position)
  Saturated normalized eR/1(normalized eR) -> Normalized eR/1
  R/1 -> "Saturated angular velocity eOmega "/3(R_cur), Saturated normalized eR/1(Current averaged rotation M)
  R_desired/1 -> "Saturated angular velocity eOmega "/4(R_desired), Saturated normalized eR/2(R_desired)
  "Saturated angular velocity eOmega "/1(Normalized angular velocity) -> "Normalized omega error "/1
  "omega_desired "/1 -> "Saturated angular velocity eOmega "/2("omega_desired ")
  "saturated normalized altitude error "/1(Position error) -> "Normalized position error "/1
  "saturated normalized altitude error "/2(velocity_error) -> Normalized velocity error/1
  "v_desired "/1 -> "saturated normalized altitude error "/4(v_desired)
  r_desired/1 -> "saturated normalized altitude error "/3("r_desired ")

== system target_driver_2022_Ctrl_v_2_4_landing_2017a/Geometric Controller/Attitude Adaptive ==
  e_R : Inport
  e_Omega : Inport  Port=2
  Enable : Inport  Port=3
  Adaptive_flag : Inport  Port=4
  adaptive_gain : Inport  Port=5
  Adaptive Control : MATLAB Function  TreatAsAtomicUnit=on
  Compare To Zero : simulink/Logic and Bit Operations/Compare To Zero  relop=>  OutDataTypeStr=uint8  ZeroCross=off
  "Integrator " : DiscreteIntegrator  InitialConditionSource=external  InitialCondition=adaptive_roll_init  SampleTime=-1  LimitOutput=on  UpperSaturationLimit=adaptive_roll_limit  LowerSaturationLimit=adaptive_roll_limit_low  ICPrevOutput=DiscIntNeverNeededParam  ICPrevScaledInput=DiscIntNeverNeededParam
  Integrator 1 : DiscreteIntegrator  InitialConditionSource=external  InitialCondition=adaptive_pitch_init  SampleTime=-1  LimitOutput=on  UpperSaturationLimit=adaptive_pitch_limit  LowerSaturationLimit=adaptive_pitch_limit_low  ICPrevOutput=DiscIntNeverNeededParam  ICPrevScaledInput=DiscIntNeverNeededParam
  Integrator 2 : DiscreteIntegrator  InitialConditionSource=external  InitialCondition=adaptive_yaw_init  SampleTime=-1  LimitOutput=on  UpperSaturationLimit=adaptive_yaw_limit  LowerSaturationLimit=adaptive_yaw_limit_low  ICPrevOutput=DiscIntNeverNeededParam  ICPrevScaledInput=DiscIntNeverNeededParam
  Mux : Mux  Inputs=3
  Product{1,5..10} (7 alike) : Product  RndMeth=Zero
  adaptive_pitch_init : Constant  Value=adaptive_pitch_init
  "adaptive_roll_init " : Constant  Value=adaptive_roll_init
  adaptive_yaw_init : Constant  Value=adaptive_yaw_init
  adaptive_roll : Outport
  adaptive_pitch : Outport  Port=2
  adaptive_yaw : Outport  Port=3
  adaptive_attitude_control : Outport  Port=4
  wires:
  Product5/1 -> "Integrator "/1
  Adaptive Control/1(der_adaptive_torque_roll) -> Product5/2
  Product6/1 -> Integrator 1/1
  Adaptive Control/2(der_adaptive_torque_pitch) -> Product6/2
  Product7/1 -> Integrator 2/1
  Product8/1 -> adaptive_roll/1
  Adaptive Control/3(der_adaptive_torque_yaw) -> Product7/2
  Product9/1 -> adaptive_pitch/1
  Product10/1 -> adaptive_yaw/1
  Adaptive_flag/1 -> Compare To Zero/1
  Compare To Zero/1 -> Product1/1, Product10/1, Product9/1, Product8/1
  Integrator 2/1 -> Mux/3, Product10/2, Adaptive Control/3(current_adaptive_yaw)
  Integrator 1/1 -> Product9/2, Adaptive Control/2(current_adaptive_pitch), Mux/2
  "Integrator "/1 -> Product8/2, Adaptive Control/1(current_adaptive_roll), Mux/1
  adaptive_gain/1 -> Adaptive Control/6(adaptive_gain_limit)
  Mux/1 -> Product1/2
  "adaptive_roll_init "/1 -> "Integrator "/2
  adaptive_pitch_init/1 -> Integrator 1/2
  adaptive_yaw_init/1 -> Integrator 2/2
  e_R/1 -> Adaptive Control/4(e_R)
  Enable/1 -> Product7/1, Product6/1, Product5/1
  e_Omega/1 -> Adaptive Control/5(e_Omega)
  Product1/1 -> adaptive_attitude_control/1

== system target_driver_2022_Ctrl_v_2_4_landing_2017a/Geometric Controller/lateral adaptive ==
  e_x : Inport
  e_v : Inport  Port=2
  Enable : Inport  Port=3
  adaptive_gain : Inport  Port=4
  Adaptive_lateral_flag : Inport  Port=5
  Adaptive Control : MATLAB Function  TreatAsAtomicUnit=on
  Compare To Zero : simulink/Logic and Bit Operations/Compare To Zero  relop=>  OutDataTypeStr=uint8  ZeroCross=off
  "Integrator " : DiscreteIntegrator  InitialConditionSource=external  InitialCondition=adaptive_roll_init  SampleTime=-1  LimitOutput=on  UpperSaturationLimit=adaptive_x_limit  LowerSaturationLimit=adaptive_x_limit_low  ICPrevOutput=DiscIntNeverNeededParam  ICPrevScaledInput=DiscIntNeverNeededParam
  Integrator 1 : DiscreteIntegrator  InitialConditionSource=external  InitialCondition=adaptive_pitch_init  SampleTime=-1  LimitOutput=on  UpperSaturationLimit=adaptive_y_limit  LowerSaturationLimit=adaptive_y_limit_low  ICPrevOutput=DiscIntNeverNeededParam  ICPrevScaledInput=DiscIntNeverNeededParam
  Integrator 2 : DiscreteIntegrator  InitialConditionSource=external  InitialCondition=adaptive_yaw_init  SampleTime=-1  LimitOutput=on  UpperSaturationLimit=adaptive_z_limit  LowerSaturationLimit=adaptive_z_limit_low  ICPrevOutput=DiscIntNeverNeededParam  ICPrevScaledInput=DiscIntNeverNeededParam
  Mux : Mux  Inputs=3
  Product{1,5..10} (7 alike) : Product  RndMeth=Zero
  "adaptive_x_init " : Constant  Value=adaptive_x_init
  adaptive_y_init : Constant  Value=adaptive_y_init
  adaptive_z_init : Constant  Value=adaptive_z_init
  adaptive_lateral_control : Outport
  adaptive_x : Outport  Port=2
  adaptive_y : Outport  Port=3
  adaptive_z : Outport  Port=4
  wires:
  Product5/1 -> "Integrator "/1
  Adaptive Control/1(der_adaptive_torque_x) -> Product5/2
  Product6/1 -> Integrator 1/1
  Adaptive Control/2(der_adaptive_torque_y) -> Product6/2
  Product7/1 -> Integrator 2/1
  Adaptive Control/3(der_adaptive_torque_z) -> Product7/2
  adaptive_gain/1 -> Adaptive Control/6(adaptive_gain_limit)
  "adaptive_x_init "/1 -> "Integrator "/2
  adaptive_y_init/1 -> Integrator 1/2
  adaptive_z_init/1 -> Integrator 2/2
  e_x/1 -> Adaptive Control/4(e_x)
  Enable/1 -> Product7/1, Product6/1, Product5/1
  e_v/1 -> Adaptive Control/5(e_v)
  Compare To Zero/1 -> Product1/1, Product10/1, Product9/1, Product8/1
  Adaptive_lateral_flag/1 -> Compare To Zero/1
  "Integrator "/1 -> Adaptive Control/1(current_adaptive_x), Product8/2, Mux/1
  Integrator 1/1 -> Adaptive Control/2(current_adaptive_y), Product9/2, Mux/2
  Product9/1 -> adaptive_y/1
  Product8/1 -> adaptive_x/1
  Integrator 2/1 -> Product10/2, Mux/3, Adaptive Control/3(current_adaptive_z)
  Product10/1 -> adaptive_z/1
  Mux/1 -> Product1/2
  Product1/1 -> adaptive_lateral_control/1

== system target_driver_2022_Ctrl_v_2_4_landing_2017a/Observer for averaged system/Attitude Observer ==
  note: Attitude averaging and filtering using geometric average in Riemannian metric SO(3)
      |
      | Patrick 2021 Mar
  Vicon Update flag : Inport
  Raw Rotation : Inport  Port=2
  Vicon Count : Inport  Port=3
  Geometric Averaging Rotation Matix : Subsystem
  Geometric derivative in SO(3) : Subsystem
  "Averaged quaternion " : Outport
  Average Rotation Matrix : Outport  Port=2
  Raw quaternion : Outport  Port=3
  Geometric filtered derivative : Outport  Port=4
  wires:
  Vicon Count/1 -> Geometric derivative in SO(3)/2(Vicon Count)
  Raw Rotation/1 -> Geometric Averaging Rotation Matix/2(Current Rotation)
  Vicon Update flag/1 -> Geometric derivative in SO(3)/4("Vicon Update Flag "), Geometric Averaging Rotation Matix/1(Vicon Update flag)
  Geometric Averaging Rotation Matix/4(Previous Averaged Rotation Matrix) -> Geometric derivative in SO(3)/1(Previous Averaged Rotation M)
  Geometric derivative in SO(3)/1(Filtered Geometric derivative in SO(3)) -> Geometric filtered derivative/1
  Geometric Averaging Rotation Matix/3("Raw quaternion output ") -> Raw quaternion/1
  Geometric Averaging Rotation Matix/1(Averaged quaternion output) -> "Averaged quaternion "/1
  Geometric Averaging Rotation Matix/2("Averaged Rotation Matrix ") -> Average Rotation Matrix/1, Geometric derivative in SO(3)/3(Current Averaged Rotation M)

== system target_driver_2022_Ctrl_v_2_4_landing_2017a/Observer for averaged system/Euler derivative & filtered angular velocity  ==
  note: The skew symmetric structure is corrected from
      | the old angular velocity calculation.
      | Note from Patrick 2021 Mar
  "Rotation matrix " : Inport
  Angular velocity : MATLAB Function  TreatAsAtomicUnit=on
  Demux : Demux  Outputs=3
  Mux : Mux  Inputs=3
  filtered derivative : Subsystem
  Angular velocity_Euler : Outport
  Frob_norm error : Outport  Port=2
  wires:
  Demux/2 -> Mux/2
  Demux/3 -> Mux/3
  Mux/1 -> Angular velocity_Euler/1
  filtered derivative/1(Out1) -> Angular velocity/2(Rdot)
  Angular velocity/1(w) -> Demux/1
  Demux/1 -> Mux/1
  Angular velocity/2(Frob_error) -> Frob_norm error/1
  "Rotation matrix "/1 -> Angular velocity/1(R), filtered derivative/1(In1)

== system target_driver_2022_Ctrl_v_2_4_landing_2017a/Observer for averaged system/Position Observer ==
  "raw_position " : Inport
  vicon Update : Inport  Port=2
  Vicon Count : Inport  Port=3
  "Averaging position & velocity " : MATLAB Function  TreatAsAtomicUnit=on
  Delay10 : Delay  DelayLength=delay(2)  InitialCondition=0
  Delay11 : Delay  DelayLength=delay(3)  InitialCondition=0
  Delay14 : Delay  DelayLength=delay(4)  InitialCondition=0
  LowPassFiltere1 : Subsystem
  LowPassFiltere2 : Subsystem
  previous position : Delay  DelayLength=1  InitialCondition=0
  previous velocity : Delay  DelayLength=1  InitialCondition=0
  Average and filtered position : Outport
  Averaged and filtered velocity : Outport  Port=2
  wires:
  previous velocity/1 -> "Averaging position & velocity "/8(vout_prev)
  "Averaging position & velocity "/2(vout) -> previous velocity/1, LowPassFiltere2/1(In1)
  previous position/1 -> "Averaging position & velocity "/7(rout_prev)
  "raw_position "/1 -> "Averaging position & velocity "/4(r_cur), Delay14/1, Delay11/1, Delay10/1
  Delay14/1 -> "Averaging position & velocity "/3(r_prev3)
  Delay11/1 -> "Averaging position & velocity "/2(r_prev2)
  Delay10/1 -> "Averaging position & velocity "/1(r_prev)
  LowPassFiltere2/1(Out1) -> Averaged and filtered velocity/1
  "Averaging position & velocity "/1(rout) -> previous position/1, LowPassFiltere1/1(In1)
  LowPassFiltere1/1(Out1) -> Average and filtered position/1
  vicon Update/1 -> "Averaging position & velocity "/5(update)
  Vicon Count/1 -> "Averaging position & velocity "/6(count)

== system target_driver_2022_Ctrl_v_2_4_landing_2017a/Observer for averaged system1/Attitude Observer ==
  note: Attitude averaging and filtering using geometric average in Riemannian metric SO(3)
      |
      | Patrick 2021 Mar
  Vicon Update flag : Inport
  Raw Rotation : Inport  Port=2
  Vicon Count : Inport  Port=3
  Geometric Averaging Rotation Matix : Subsystem
  Geometric derivative in SO(3) : Subsystem
  "Averaged quaternion " : Outport
  Average Rotation Matrix : Outport  Port=2
  Raw quaternion : Outport  Port=3
  Geometric filtered derivative : Outport  Port=4
  wires:
  Vicon Count/1 -> Geometric derivative in SO(3)/2(Vicon Count)
  Raw Rotation/1 -> Geometric Averaging Rotation Matix/2(Current Rotation)
  Vicon Update flag/1 -> Geometric derivative in SO(3)/4("Vicon Update Flag "), Geometric Averaging Rotation Matix/1(Vicon Update flag)
  Geometric Averaging Rotation Matix/4(Previous Averaged Rotation Matrix) -> Geometric derivative in SO(3)/1(Previous Averaged Rotation M)
  Geometric derivative in SO(3)/1(Filtered Geometric derivative in SO(3)) -> Geometric filtered derivative/1
  Geometric Averaging Rotation Matix/3("Raw quaternion output ") -> Raw quaternion/1
  Geometric Averaging Rotation Matix/1(Averaged quaternion output) -> "Averaged quaternion "/1
  Geometric Averaging Rotation Matix/2("Averaged Rotation Matrix ") -> Average Rotation Matrix/1, Geometric derivative in SO(3)/3(Current Averaged Rotation M)

== system target_driver_2022_Ctrl_v_2_4_landing_2017a/Observer for averaged system1/Euler derivative & filtered angular velocity  ==
  note: The skew symmetric structure is corrected from
      | the old angular velocity calculation.
      | Note from Patrick 2021 Mar
  "Rotation matrix " : Inport
  Angular velocity : MATLAB Function  TreatAsAtomicUnit=on
  Demux : Demux  Outputs=3
  Mux : Mux  Inputs=3
  filtered derivative : Subsystem
  Angular velocity_Euler : Outport
  Frob_norm error : Outport  Port=2
  wires:
  Demux/2 -> Mux/2
  Demux/3 -> Mux/3
  Mux/1 -> Angular velocity_Euler/1
  filtered derivative/1(Out1) -> Angular velocity/2(Rdot)
  Angular velocity/1(w) -> Demux/1
  Demux/1 -> Mux/1
  Angular velocity/2(Frob_error) -> Frob_norm error/1
  "Rotation matrix "/1 -> Angular velocity/1(R), filtered derivative/1(In1)

== system target_driver_2022_Ctrl_v_2_4_landing_2017a/Observer for averaged system1/Position Observer ==
  "raw_position " : Inport
  vicon Update : Inport  Port=2
  Vicon Count : Inport  Port=3
  "Averaging position & velocity " : MATLAB Function  TreatAsAtomicUnit=on
  Delay10 : Delay  DelayLength=delay(2)  InitialCondition=0
  Delay11 : Delay  DelayLength=delay(3)  InitialCondition=0
  Delay14 : Delay  DelayLength=delay(4)  InitialCondition=0
  LowPassFiltere1 : Subsystem
  LowPassFiltere2 : Subsystem
  previous position : Delay  DelayLength=1  InitialCondition=0
  previous velocity : Delay  DelayLength=1  InitialCondition=0
  Average and filtered position : Outport
  Averaged and filtered velocity : Outport  Port=2
  wires:
  previous velocity/1 -> "Averaging position & velocity "/8(vout_prev)
  "Averaging position & velocity "/2(vout) -> previous velocity/1, LowPassFiltere2/1(In1)
  previous position/1 -> "Averaging position & velocity "/7(rout_prev)
  "raw_position "/1 -> "Averaging position & velocity "/4(r_cur), Delay14/1, Delay11/1, Delay10/1
  Delay14/1 -> "Averaging position & velocity "/3(r_prev3)
  Delay11/1 -> "Averaging position & velocity "/2(r_prev2)
  Delay10/1 -> "Averaging position & velocity "/1(r_prev)
  LowPassFiltere2/1(Out1) -> Averaged and filtered velocity/1
  "Averaging position & velocity "/1(rout) -> previous position/1, LowPassFiltere1/1(In1)
  LowPassFiltere1/1(Out1) -> Average and filtered position/1
  vicon Update/1 -> "Averaging position & velocity "/5(update)
  Vicon Count/1 -> "Averaging position & velocity "/6(count)

== system target_driver_2022_Ctrl_v_2_4_landing_2017a/Open_Closed_loop_selection/SIgnalForRamp_binary ==
  note: Should output 1 or -1,
      | so signal ramps UP to 1
      | or DOWN to 0.
  In1 : Inport
  Add : Sum  Inputs=+-
  Compare To Zero : simulink/Logic and Bit Operations/Compare To Zero  relop=>  OutDataTypeStr=uint8  ZeroCross=off
  Constant : Constant
  Data Type Conversion : DataTypeConversion  OutDataTypeStr=double  SaturateOnIntegerOverflow=off  RndMeth=Floor
  Gain : Gain  Gain=2
  Out1 : Outport
  wires:
  In1/1 -> Compare To Zero/1
  Compare To Zero/1 -> Data Type Conversion/1
  Gain/1 -> Add/1
  Constant/1 -> Add/2
  Add/1 -> Out1/1
  Data Type Conversion/1 -> Gain/1

== system target_driver_2022_Ctrl_v_2_4_landing_2017a/Open_Closed_loop_selection/counter ==
  running time : Inport
  Add : Sum  Inputs=+-
  Compare To Zero : simulink/Logic and Bit Operations/Compare To Zero  relop=<  OutDataTypeStr=uint8  ZeroCross=off
  Product2 : Product  RndMeth=Zero
  SaturatingRamp : DiscreteIntegrator  gainval=1  SampleTime=-1  UpperSaturationLimit=1  LowerSaturationLimit=0  ICPrevOutput=DiscIntNeverNeededParam  ICPrevScaledInput=DiscIntNeverNeededParam
  constant : Constant
  start delay compare : simulink/Logic and Bit Operations/Compare To Constant  relop=>  const=start_delay  OutDataTypeStr=uint8
  enable : Outport
  wires:
  SaturatingRamp/1 -> Add/1, start delay compare/1
  running time/1 -> Add/2
  Add/1 -> Compare To Zero/1
  start delay compare/1 -> Product2/1
  Compare To Zero/1 -> Product2/2
  Product2/1 -> enable/1
  constant/1 -> SaturatingRamp/1

== system target_driver_2022_Ctrl_v_2_4_landing_2017a/Open_Closed_loop_selection/counter1 ==
  running time : Inport
  Add : Sum  Inputs=+-
  Compare To Zero : simulink/Logic and Bit Operations/Compare To Zero  relop=<  OutDataTypeStr=uint8  ZeroCross=off
  Product2 : Product  RndMeth=Zero
  SaturatingRamp : DiscreteIntegrator  gainval=1  SampleTime=-1  UpperSaturationLimit=1  LowerSaturationLimit=0  ICPrevOutput=DiscIntNeverNeededParam  ICPrevScaledInput=DiscIntNeverNeededParam
  constant : Constant
  start control delay compare : simulink/Logic and Bit Operations/Compare To Constant  relop=>  const=start_delay_control  OutDataTypeStr=uint8
  enable : Outport
  wires:
  SaturatingRamp/1 -> Add/1, start control delay compare/1
  running time/1 -> Add/2
  Add/1 -> Compare To Zero/1
  start control delay compare/1 -> Product2/1
  Compare To Zero/1 -> Product2/2
  Product2/1 -> enable/1
  constant/1 -> SaturatingRamp/1

== system target_driver_2022_Ctrl_v_2_4_landing_2017a/Open_Closed_loop_selection/timer1 ==
  SaturatingRamp : DiscreteIntegrator  gainval=1  SampleTime=-1  UpperSaturationLimit=1  LowerSaturationLimit=0  ICPrevOutput=DiscIntNeverNeededParam  ICPrevScaledInput=DiscIntNeverNeededParam
  constant : Constant
  time : Outport
  wires:
  SaturatingRamp/1 -> time/1
  constant/1 -> SaturatingRamp/1

== system target_driver_2022_Ctrl_v_2_4_landing_2017a/Phantom1/timer1 ==
  SaturatingRamp : DiscreteIntegrator  gainval=1  SampleTime=-1  UpperSaturationLimit=1  LowerSaturationLimit=0  ICPrevOutput=DiscIntNeverNeededParam  ICPrevScaledInput=DiscIntNeverNeededParam
  constant : Constant
  time : Outport
  wires:
  SaturatingRamp/1 -> time/1
  constant/1 -> SaturatingRamp/1
